simulink subsystem "samplemodel_plotLookupTable1DBlocks_refsub"  (R2025b)
settings: Solver=VariableStepAuto  StartTime=0.0  StopTime=10.0  RelTol=1e-3
libraries: fl_lib x8, simulink x1
settings Model: Creator=isaacito  LastModifiedBy=isaacito

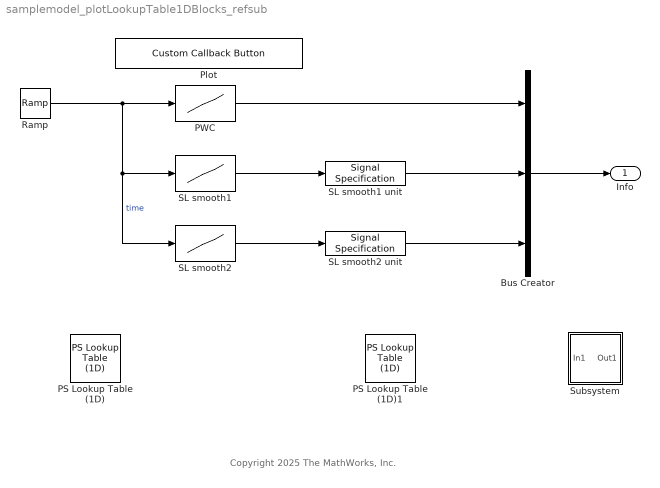
== system samplemodel_plotLookupTable1DBlocks_refsub ==
  note: Copyright 2025 The MathWorks, Inc.
  Bus Creator : BusCreator  Inputs=3
  PS Lookup Table (1D) : fl_lib/Physical Signals/Lookup Tables/PS Lookup Table (1D)  x=[0 1 2 5 6 7]  f=[0 1 -1 0 -1 1]  interp_method=simscape.enum.interpolation.linear  extrap_method=simscape.enum.extrapolation.linear
      settings: AttributesFormatString=|
      | interp_method: %<interp_method>
      | extrap_method: %<extrap_method>
      | f_unit: %<f_unit>
      | x_unit: %<x_unit>
  PS Lookup Table (1D)1 : fl_lib/Physical Signals/Lookup Tables/PS Lookup Table (1D)  x=[0 1 2 5 6 7] s  f=[2 2 2 4 4 4]  interp_method=simscape.enum.interpolation.smooth  extrap_method=simscape.enum.extrapolation.nearest
      settings: AttributesFormatString=|
      | interp_method: %<interp_method>
      | extrap_method: %<extrap_method>
      | f_unit: %<f_unit>
      | x_unit: %<x_unit>
  PWC : Lookup_n-D  NumberOfTableDimensions=1  BreakpointsForDimension1=[0, 3, 5]  Table=[0, 2, 1]  InterpMethod=Flat  InternalRulePriority=Speed  RndMeth=Simplest
  Plot : CustomCallbackButton  Configuration="{\"components\":[{\"name\":\"BackgroundImageComponent\",\"settings\":{\"image\":{\"size\":[0,0],\"src\":\"default\",\"srcOrientation\":\"Right\"},\"position\":[0,0,1,1]}},{\"name\":\"ButtonStateComponent\",\"settings\":{\"buttonType\":\"momentary\",\"clickFcn\":\"ModelUtil1.plotLookupTable1DBlocks(gcs, SearchDepth=1, Blocks=[\\\"PWC\\\" \\\"SL smooth1\\\" \\\"SL smooth2\\\" \\\"PS Lookup Table (1D)\\\" \\\"PS Lookup Table (1D)1\\\"])\",\"onValue\":1,\"position\":[0,0,1,1],\"pressDelay\":\"500\",\"pressFcn\":\"\",\"repeatInterval\":\"0\",\"states\":[{\"horizontalAlignment\":\"center\",\"image\":{\"position\":[0,0,1,1],\"size\":[1,1],\"src\":\"default\",\"srcOrientation\":\"Right\"},\"label\":{\"color\":[0.01176470588,0.01176470588,0.01176470588,1],\"icon\":{\"size\":[0,0],\"src\":\"default\",\"srcOrientation\":\"Right\"},\"iconOffset\":0,\"iconPlacement\":\"left\",\"opacity\":1,\"show\":true,\"text\":{\"content\":\"Lookup table 1D blocks\",\"font\":\"Helvetica\"}},\"labelOffset\":[0,0],\"verticalAlignment\":\"middle\"},{\"horizontalAlignment\":\"center\",\"image\":{\"position\":[0,0,1,1],\"size\":[1,1],\"src\":\"default\",\"srcOrientation\":\"Right\"},\"label\":{\"color\":[0.01176470588,0.01176470588,0.01176470588,1],\"icon\":{\"size\":[0,0],\"src\":\"default\",\"srcOrientation\":\"Right\"},\"iconOffset\":0,\"iconPlacement\":\"left\",\"opacity\":1,\"show\":true,\"text\":{\"content\":\"Lookup table 1D blocks\",\"font\":\"Helvetica\"}},\"labelOffset\":[0,0],\"verticalAlignment\":\"middle\"},{\"horizontalAlignment\":\"center\",\"image\":{\"position\":[0,0,1,1],\"size\":[1,1],\"src\":\"default\",\"srcOrientation\":\"Right\"},\"label\":{\"color\":[0.01176470588,0.01176470588,0.01176470588,1],\"icon\":{\"size\":[0,0],\"src\":\"default\",\"srcOrientation\":\"Right\"},\"iconOffset\":0,\"iconPlacement\":\"left\",\"opacity\":1,\"show\":true,\"text\":{\"content\":\"Lookup table 1D blocks\",\"font\":\"Helvetica\"}},\"labelOffset\":[0,0],\"verticalAlignment\":\"middle\"},{\"horizontalAlignment\":\"center\",\"image\":{\"position\":[0,0,1,1],\"size\":[1,1],\"src\":\"default\",\"srcOrientation\":\"Right\"},\"label\":{\"color\":[0.01176470588,0.01176470588,0.01176470588,1],\"icon\":{\"size\":[0,0],\"src\":\"default\",\"srcOrientation\":\"Right\"},\"iconOffset\":0,\"iconPlacement\":\"left\",\"opacity\":1,\"show\":true,\"text\":{\"content\":\"Lookup table 1D blocks\",\"font\":\"Helvetica\"}},\"labelOffset\":[0,0],\"verticalAlignment\":\"middle\"}]}},{\"name\":\"ForegroundImageComponent\",\"settings\":{\"image\":{\"size\":[0,0],\"src\":\"default\",\"srcOrientation\":\"Right\"},\"isForeground\":1,\"position\":[0,0,1,1]}}],\"derived\":{\"blockParameters\":{\"AutoActivate\":true,\"ButtonText\":\"Lookup table 1D blocks\",\"ButtonType\":\"Momentary\",\"ClickFcn\":\"ModelUtil1.plotLookupTable1DBlocks(gcs, SearchDepth=1, Blocks=[\\\"PWC\\\" \\\"SL smooth1\\\" \\\"SL smooth2\\\" \\\"PS Lookup Table (1D)\\\" \\\"PS Lookup Table (1D)1\\\"])\",\"OnValue\":1,\"PressDelay\":\"500\",\"PressFcn\":\"\",\"RepeatInterval\":\"0\",\"fixedAspectRatio\":\"off\"}},\"settings\":{\"BindingType\":\"standalone\",\"autoActivate\":true,\"backgroundColor\":[244,244,244,1],\"backgroundOffset\":0.2,\"backgroundOpacity\":1,\"fixedAspectRatio\":\"off\",\"foregroundColor\":[0.01176470588,0.01176470588,0.01176470588,1],\"migratedFromLegacy\":true,\"useBackgroundColor\":true,\"variant\":\"callback\",\"version\":\"R2025a\"},\"type\":\"Button\"}"  CustomBackgroundColor="{\"color\":[0.9568627451,0.9568627451,0.9568627451],\"show\":true}"
  Ramp : simulink/Sources/Ramp  slope=1  start=0  InitialOutput=0
      settings: AttributesFormatString=|
      | Slope: %<slope>
      | Start time: %<start>
      | Initial output: %<InitialOutput>
  SL smooth1 : Lookup_n-D  NumberOfTableDimensions=1  BreakpointsForDimension1=[0 1 2 3 5 6 7]  Table=[0 0 0 2 1 1 1]  InterpMethod=Akima spline  InternalRulePriority=Speed  RndMeth=Simplest
  SL smooth1 unit : SignalSpecification  Unit=rpm
  SL smooth2 : Lookup_n-D  NumberOfTableDimensions=1  BreakpointsForDimension1=[0 1 3 5 6 7]  Table=[0 1 0 -1 0 1]  InterpMethod=Akima spline  InternalRulePriority=Speed  RndMeth=Simplest
  SL smooth2 unit : SignalSpecification  Unit=N*m
  Subsystem : Subsystem
  Info : Outport
  wires:
  SL smooth2/1 -> SL smooth2 unit/1
  SL smooth1/1 -> SL smooth1 unit/1
  Ramp/1 -> PWC/1, SL smooth2/1, SL smooth1/1  "time"
  PWC/1 -> Bus Creator/1
  SL smooth1 unit/1 -> Bus Creator/2
  SL smooth2 unit/1 -> Bus Creator/3
  Bus Creator/1 -> Info/1

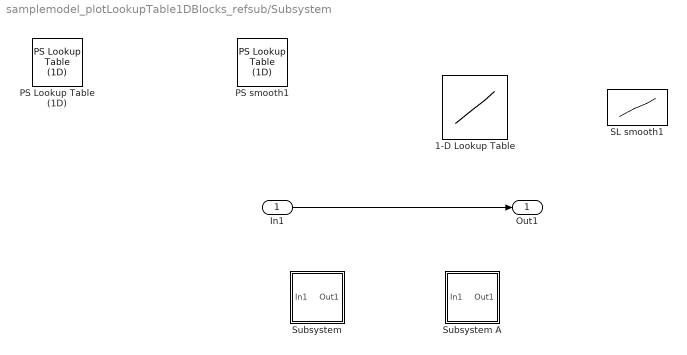
== system samplemodel_plotLookupTable1DBlocks_refsub/Subsystem ==
  In1 : Inport
  1-D Lookup Table : Lookup_n-D  NumberOfTableDimensions=1  BreakpointsForDimension1=[-5:5]  Table=tanh([-5:5])  InternalRulePriority=Speed  RndMeth=Simplest
  PS Lookup Table (1D) : fl_lib/Physical Signals/Lookup Tables/PS Lookup Table (1D)  x=[1, 2, 3, 4, 5]  f=[0, 1, 2, 3, 4]  interp_method=simscape.enum.interpolation.linear  extrap_method=simscape.enum.extrapolation.linear
  PS smooth1 : fl_lib/Physical Signals/Lookup Tables/PS Lookup Table (1D)  x=[0 1 2 5 6 7] s  f=[2 3 0 0 4 4]  interp_method=simscape.enum.interpolation.smooth  extrap_method=simscape.enum.extrapolation.nearest
      settings: AttributesFormatString=|
      | interp_method: %<interp_method>
      | extrap_method: %<extrap_method>
      | f_unit: %<f_unit>
      | x_unit: %<x_unit>
  SL smooth1 : Lookup_n-D  NumberOfTableDimensions=1  BreakpointsForDimension1=[0 1 2 5 6 7]  Table=[2 3 0 0 4 4]  InterpMethod=Akima spline  InternalRulePriority=Speed  RndMeth=Simplest
  Subsystem : Subsystem
  Subsystem A : Subsystem
  Out1 : Outport
  wires:
  In1/1 -> Out1/1

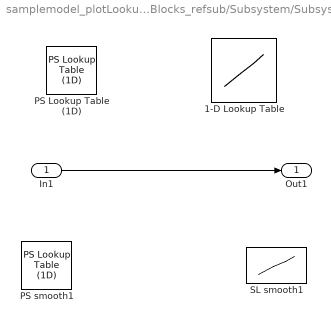
== system samplemodel_plotLookupTable1DBlocks_refsub/Subsystem/Subsystem ==
  In1 : Inport
  1-D Lookup Table : Lookup_n-D  NumberOfTableDimensions=1  BreakpointsForDimension1=[-5:5]  Table=tanh([-5:5])  InternalRulePriority=Speed  RndMeth=Simplest
  PS Lookup Table (1D) : fl_lib/Physical Signals/Lookup Tables/PS Lookup Table (1D)  x=[1, 2, 3, 4, 5]  f=[0, 1, 2, 3, 4]  interp_method=simscape.enum.interpolation.linear  extrap_method=simscape.enum.extrapolation.linear
  PS smooth1 : fl_lib/Physical Signals/Lookup Tables/PS Lookup Table (1D)  x=[0 1 2 5 6 7] s  f=[-2 -3 0 0 -4 -4]  interp_method=simscape.enum.interpolation.smooth  extrap_method=simscape.enum.extrapolation.nearest
      settings: AttributesFormatString=|
      | interp_method: %<interp_method>
      | extrap_method: %<extrap_method>
      | f_unit: %<f_unit>
      | x_unit: %<x_unit>
  SL smooth1 : Lookup_n-D  NumberOfTableDimensions=1  BreakpointsForDimension1=[0 1 2 5 6 7]  Table=[-2 -3 0 0 -4 -4]  InterpMethod=Akima spline  InternalRulePriority=Speed  RndMeth=Simplest
  Out1 : Outport
  wires:
  In1/1 -> Out1/1

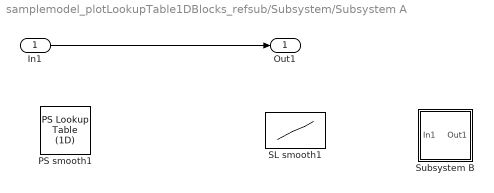
== system samplemodel_plotLookupTable1DBlocks_refsub/Subsystem/Subsystem A ==
  In1 : Inport
  PS smooth1 : fl_lib/Physical Signals/Lookup Tables/PS Lookup Table (1D)  x=[0 1 2 5 6 7] s  f=[3 2 0 0 0 4] N*m  interp_method=simscape.enum.interpolation.smooth  extrap_method=simscape.enum.extrapolation.nearest
      settings: AttributesFormatString=|
      | interp_method: %<interp_method>
      | extrap_method: %<extrap_method>
      | f_unit: %<f_unit>
      | x_unit: %<x_unit>
  SL smooth1 : Lookup_n-D  NumberOfTableDimensions=1  BreakpointsForDimension1=[0 1 2 5 6 7]  Table=[3 2 0 0 0 4]  InterpMethod=Akima spline  InternalRulePriority=Speed  RndMeth=Simplest
  Subsystem B : Subsystem
  Out1 : Outport
  wires:
  In1/1 -> Out1/1

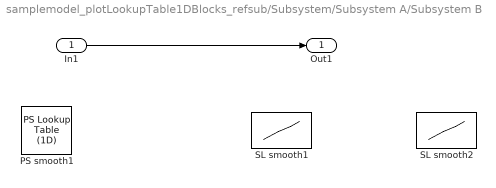
== system samplemodel_plotLookupTable1DBlocks_refsub/Subsystem/Subsystem A/Subsystem B ==
  In1 : Inport
  PS smooth1 : fl_lib/Physical Signals/Lookup Tables/PS Lookup Table (1D)  x=[0 1 2 4 5 6 7] s  f="[3 3 3  0 1 1 1]"  interp_method=simscape.enum.interpolation.smooth  extrap_method=simscape.enum.extrapolation.nearest
      settings: AttributesFormatString=|
      | interp_method: %<interp_method>
      | extrap_method: %<extrap_method>
      | f_unit: %<f_unit>
      | x_unit: %<x_unit>
  SL smooth1 : Lookup_n-D  NumberOfTableDimensions=1  BreakpointsForDimension1=[0 1 2 4 5 6 7]  Table="[3 3 3  0 1 1 1]"  InterpMethod=Akima spline  InternalRulePriority=Speed  RndMeth=Simplest
  SL smooth2 : Lookup_n-D  NumberOfTableDimensions=1  BreakpointsForDimension1=[0 1 2 4 5 6 7]  Table="[3 3 3  0 1 1 1]"  InterpMethod=Akima spline  InternalRulePriority=Speed  RndMeth=Simplest
  Out1 : Outport
  wires:
  In1/1 -> Out1/1
